simulink model "QuadcopterSimulationControl"  (R2016b)
settings: Solver=VariableStepAuto  StartTime=0.0  StopTime=100  RelTol=1e-3
values from neighbouring files (symbols this model uses):
  Ax = 0.1    [QuadcopterContants.m]
  Ay = 0.1    [QuadcopterContants.m]
  Az = 0.1    [QuadcopterContants.m]
  b = 1.144e-8    (= 1.144e-08)    [QuadcopterContants.m]
  d = 9.94e-10    [QuadcopterContants.m]
  g = 9.81    [QuadcopterContants.m]
  Ixx = 4.856e-3    (= 0.004856)    [QuadcopterContants.m]
  Iyy = 4.856e-3    (= 0.004856)    [QuadcopterContants.m]
  Izz = 8.801e-3    (= 0.008801)    [QuadcopterContants.m]
  Jr = 3.357e-5    (= 3.357e-05)    [QuadcopterContants.m]
  K_phi_D = 1    [QuadcopterContants.m]
  K_phi_I = 1    [QuadcopterContants.m]
  K_phi_p = 1    [QuadcopterContants.m]
  K_psi_D = 1    [QuadcopterContants.m]
  K_psi_I = 1    [QuadcopterContants.m]
  K_psi_p = 1    [QuadcopterContants.m]
  K_theta_D = 1    [QuadcopterContants.m]
  K_theta_I = 1    [QuadcopterContants.m]
  K_theta_p = 1    [QuadcopterContants.m]
  K_z_D = 1    [QuadcopterContants.m]
  K_z_I = 1    [QuadcopterContants.m]
  K_z_p = 1    [QuadcopterContants.m]
  l = 0.225    [QuadcopterContants.m]
  m = 0.468    [QuadcopterContants.m]
settings Model: Creator=alexzongo  LastModifiedBy=alexzongo

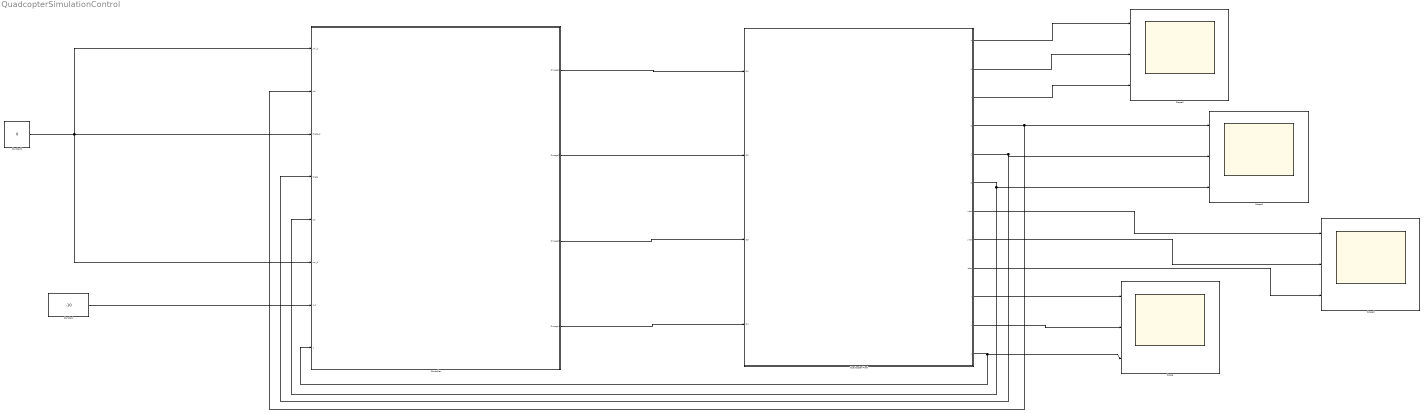
== system QuadcopterSimulationControl ==
  Constant : Constant  Value=-10
  Constant1 : Constant  Value=0
  Controller : Subsystem
  Quadcopter Plant : Subsystem
  Scope{,1..3} (4 alike) : Scope  NumInputPorts=3
  wires:
  Quadcopter Plant/4(𝜙) -> Scope1/1, Controller/2(phi)
  Quadcopter Plant/5("𝜃 ") -> Scope1/2, Controller/4(theta)
  Quadcopter Plant/6(𝜓) -> Scope1/3, Controller/5(psi)
  Quadcopter Plant/12(z) -> Scope/3, Controller/8(z)
  Controller/1(Omega1) -> Quadcopter Plant/1(Ω1)
  Controller/2(Omega2) -> Quadcopter Plant/2("Ω2 ")
  Controller/3(Omega3) -> Quadcopter Plant/3(Ω3)
  Controller/4(Omega4) -> Quadcopter Plant/4(Ω4)
  Constant1/1 -> Controller/6(psi_d), Controller/1(phi_d), Controller/3(theta_d)
  Constant/1 -> Controller/7(z_d)
  Quadcopter Plant/10(x) -> Scope/1
  Quadcopter Plant/11(y) -> Scope/2
  Quadcopter Plant/1(p) -> Scope2/1
  Quadcopter Plant/2(q) -> Scope2/2
  Quadcopter Plant/3(r) -> Scope2/3
  Quadcopter Plant/7(xdot) -> Scope3/1
  Quadcopter Plant/8(ydot) -> Scope3/2
  Quadcopter Plant/9(zdot) -> Scope3/3

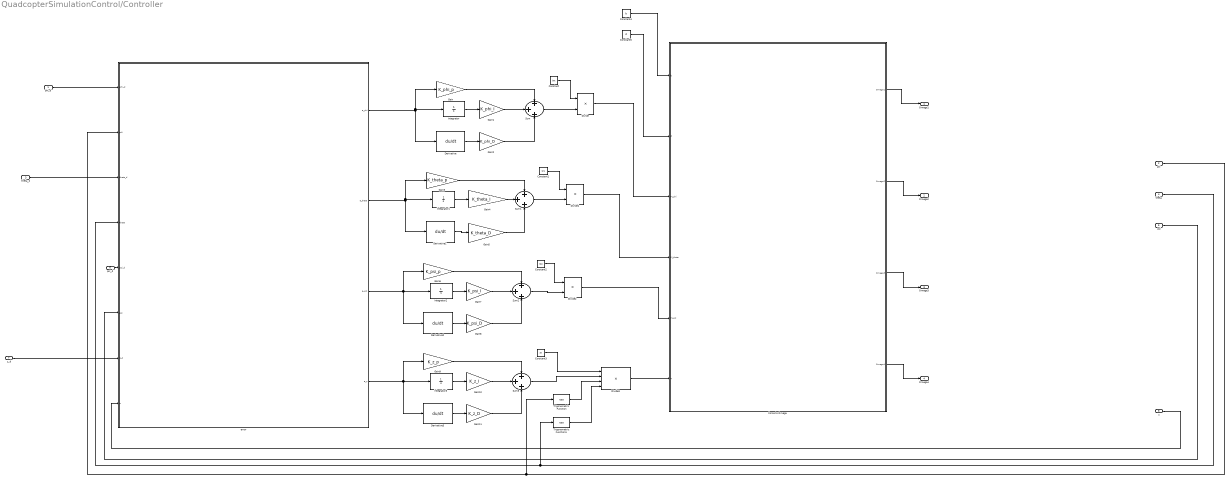
== system QuadcopterSimulationControl/Controller ==
  phi_d : Inport
  phi : Inport  Port=2
  theta_d : Inport  Port=3
  theta : Inport  Port=4
  psi : Inport  Port=5
  psi_d : Inport  Port=6
  z_d : Inport  Port=7
  z : Inport  Port=8
  Constant : Constant  Value=Ixx
  Constant1 : Constant  Value=Iyy
  Constant2 : Constant  Value=Izz
  Constant3 : Constant  Value=m
  Constant4 : Constant  Value=b
  Constant5 : Constant  Value=d
  Derivative{,1..3} (4 alike) : Derivative  CoefficientInTFapproximation=0
  Divide : Product  Inputs=**
  Divide1 : Product  Inputs=**
  Divide2 : Product  Inputs=**
  Divide3 : Product  Inputs=****
  Force to Omega : MATLAB Function  TreatAsAtomicUnit=on
  Gain : Gain  Gain=K_phi_p
  Gain1 : Gain  Gain=K_phi_I
  Gain10 : Gain  Gain=K_z_I
  Gain11 : Gain  Gain=K_z_D
  Gain2 : Gain  Gain=K_phi_D
  Gain3 : Gain  Gain=K_theta_p
  Gain4 : Gain  Gain=K_theta_I
  Gain5 : Gain  Gain=K_theta_D
  Gain6 : Gain  Gain=K_psi_p
  Gain7 : Gain  Gain=K_psi_I
  Gain8 : Gain  Gain=K_psi_D
  Gain9 : Gain  Gain=K_z_p
  Integrator{,1..3} (4 alike) : Integrator
  Sum{,1..3} (4 alike) : Sum  Inputs=+++
  Trigonometric Function : Trigonometry  Operator=cos
  Trigonometric Function1 : Trigonometry  Operator=cos
  error : MATLAB Function  TreatAsAtomicUnit=on
  Omega1 : Outport
  Omega2 : Outport  Port=2
  Omega3 : Outport  Port=3
  Omega4 : Outport  Port=4
  wires:
  Constant2/1 -> Divide2/1
  Divide2/1 -> Force to Omega/5(M_psi)
  Gain8/1 -> Sum2/3
  Constant3/1 -> Divide3/1
  Divide3/1 -> Force to Omega/6(T)
  Gain7/1 -> Sum2/2
  Sum2/1 -> Divide2/2
  Gain6/1 -> Sum2/1
  Derivative3/1 -> Gain11/1
  Gain10/1 -> Sum3/2
  Sum3/1 -> Divide3/2
  Gain11/1 -> Sum3/3
  Force to Omega/1(Omega1) -> Omega1/1
  Gain9/1 -> Sum3/1
  Force to Omega/4(Omega4) -> Omega4/1
  z_d/1 -> error/7(z_d)
  Derivative/1 -> Gain2/1
  Integrator/1 -> Gain1/1
  Divide/1 -> Force to Omega/3(M_phi)
  theta_d/1 -> error/3(theta_d)
  Gain1/1 -> Sum/2
  Gain/1 -> Sum/1
  error/1(e_phi) -> Derivative/1, Gain/1, Integrator/1
  phi/1 -> Trigonometric Function/1, error/2(phi)
  Trigonometric Function1/1 -> Divide3/4
  psi/1 -> error/6(psi)
  phi_d/1 -> error/1(phi_d)
  theta/1 -> Trigonometric Function1/1, error/4(theta)
  error/3(e_psi) -> Derivative2/1, Gain6/1, Integrator2/1
  Integrator2/1 -> Gain7/1
  Gain2/1 -> Sum/3
  error/2(e_theta) -> Derivative1/1, Gain3/1, Integrator1/1
  Divide1/1 -> Force to Omega/4(M_theta)
  error/4(e_z) -> Derivative3/1, Gain9/1, Integrator3/1
  Constant1/1 -> Divide1/1
  Integrator3/1 -> Gain10/1
  Gain5/1 -> Sum1/3
  Sum1/1 -> Divide1/2
  Derivative1/1 -> Gain5/1
  psi_d/1 -> error/5(psi_d)
  Force to Omega/3(Omega3) -> Omega3/1
  Force to Omega/2(Omega2) -> Omega2/1
  Gain3/1 -> Sum1/1
  Trigonometric Function/1 -> Divide3/3
  Gain4/1 -> Sum1/2
  Integrator1/1 -> Gain4/1
  Derivative2/1 -> Gain8/1
  Constant/1 -> Divide/1
  z/1 -> error/8(z)
  Sum/1 -> Divide/2
  Constant4/1 -> Force to Omega/1(b)
  Constant5/1 -> Force to Omega/2(d)

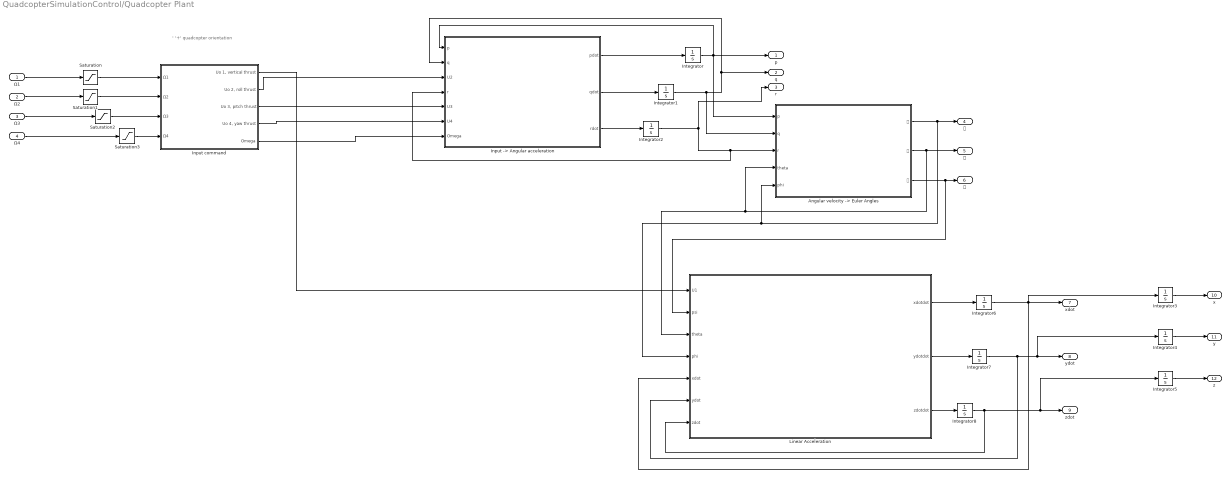
== system QuadcopterSimulationControl/Quadcopter Plant ==
  note: ' '+' quadcopter orientation
  Ω1 : Inport
  "Ω2 " : Inport  Port=2
  Ω3 : Inport  Port=3
  Ω4 : Inport  Port=4
  "Angular velocity -> Euler Angles" : Subsystem
  "Input -> Angular acceleration" : Subsystem
  "Input command " : Subsystem
  Integrator{,1..2,6..8} (6 alike) : Integrator
  Integrator3 : Integrator  LimitOutput=on
  Integrator4 : Integrator  LimitOutput=on
  Integrator5 : Integrator  LimitOutput=on  UpperSaturationLimit=0
  Linear Acceleration : Subsystem
  Saturation{,1..3} (4 alike) : Saturate  UpperLimit=inf  LowerLimit=0
  p : Outport
  q : Outport  Port=2
  r : Outport  Port=3
  𝜙 : Outport  Port=4
  "𝜃 " : Outport  Port=5
  𝜓 : Outport  Port=6
  xdot : Outport  Port=7
  ydot : Outport  Port=8
  zdot : Outport  Port=9
  x : Outport  Port=10
  y : Outport  Port=11
  z : Outport  Port=12
  wires:
  Ω1/1 -> Saturation/1
  "Ω2 "/1 -> Saturation1/1
  Ω3/1 -> Saturation2/1
  Ω4/1 -> Saturation3/1
  "Input command "/1("Uo 1, vertical thrust") -> Linear Acceleration/1(U1)
  Integrator/1 -> "Angular velocity -> Euler Angles"/1(p), "Input -> Angular acceleration"/1(p), p/1
  Integrator1/1 -> q/1, "Input -> Angular acceleration"/2(q), "Angular velocity -> Euler Angles"/2(q)
  Integrator2/1 -> r/1, "Input -> Angular acceleration"/4(r), "Angular velocity -> Euler Angles"/3(r)
  Integrator8/1 -> Integrator5/1, zdot/1, Linear Acceleration/7(zdot)
  Integrator7/1 -> Linear Acceleration/6(ydot), Integrator4/1, ydot/1
  Integrator6/1 -> Integrator3/1, Linear Acceleration/5(xdot), xdot/1
  "Input command "/2("Uo 2, roll thrust") -> "Input -> Angular acceleration"/3(U2)
  "Input command "/3("Uo 3, pitch thrust") -> "Input -> Angular acceleration"/5(U3)
  "Input command "/5(Omega) -> "Input -> Angular acceleration"/7(Omega)
  "Input -> Angular acceleration"/1(pdot) -> Integrator/1
  "Input -> Angular acceleration"/2(qdot) -> Integrator1/1
  "Input -> Angular acceleration"/3(rdot) -> Integrator2/1
  "Angular velocity -> Euler Angles"/3(𝜓) -> Linear Acceleration/2(psi), 𝜓/1
  "Angular velocity -> Euler Angles"/1(𝜙) -> Linear Acceleration/4(phi), "Angular velocity -> Euler Angles"/5(phi), 𝜙/1
  "Angular velocity -> Euler Angles"/2(𝜃) -> Linear Acceleration/3(theta), "Angular velocity -> Euler Angles"/4(theta), "𝜃 "/1
  Linear Acceleration/1(xdotdot) -> Integrator6/1
  Linear Acceleration/2(ydotdot) -> Integrator7/1
  Linear Acceleration/3(zdotdot) -> Integrator8/1
  Integrator3/1 -> x/1
  Integrator4/1 -> y/1
  Integrator5/1 -> z/1
  Saturation/1 -> "Input command "/1(Ω1)
  Saturation1/1 -> "Input command "/2("Ω2 ")
  Saturation2/1 -> "Input command "/3(Ω3)
  Saturation3/1 -> "Input command "/4(Ω4)
  "Input command "/4("Uo 4, yaw thrust") -> "Input -> Angular acceleration"/6(U4)

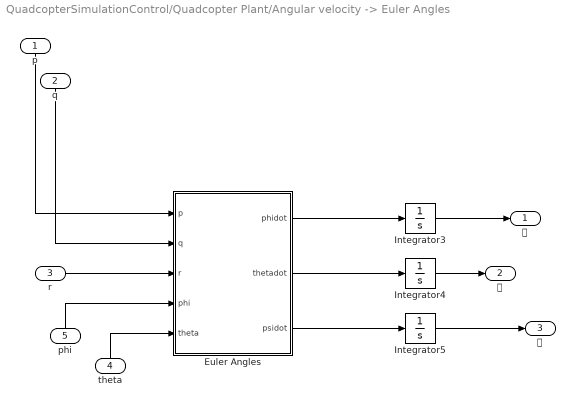
== system QuadcopterSimulationControl/Quadcopter Plant/Angular velocity -> Euler Angles ==
  p : Inport
  q : Inport  Port=2
  r : Inport  Port=3
  theta : Inport  Port=4
  phi : Inport  Port=5
  Euler Angles : MATLAB Function  TreatAsAtomicUnit=on
  Integrator3 : Integrator  WrapState=on
  Integrator4 : Integrator  WrapState=on
  Integrator5 : Integrator  WrapState=on
  𝜙 : Outport
  𝜃 : Outport  Port=2
  𝜓 : Outport  Port=3
  wires:
  theta/1 -> Euler Angles/5(theta)
  p/1 -> Euler Angles/1(p)
  phi/1 -> Euler Angles/4(phi)
  q/1 -> Euler Angles/2(q)
  r/1 -> Euler Angles/3(r)
  Euler Angles/3(psidot) -> Integrator5/1
  Integrator3/1 -> 𝜙/1
  Euler Angles/2(thetadot) -> Integrator4/1
  Integrator5/1 -> 𝜓/1
  Euler Angles/1(phidot) -> Integrator3/1
  Integrator4/1 -> 𝜃/1

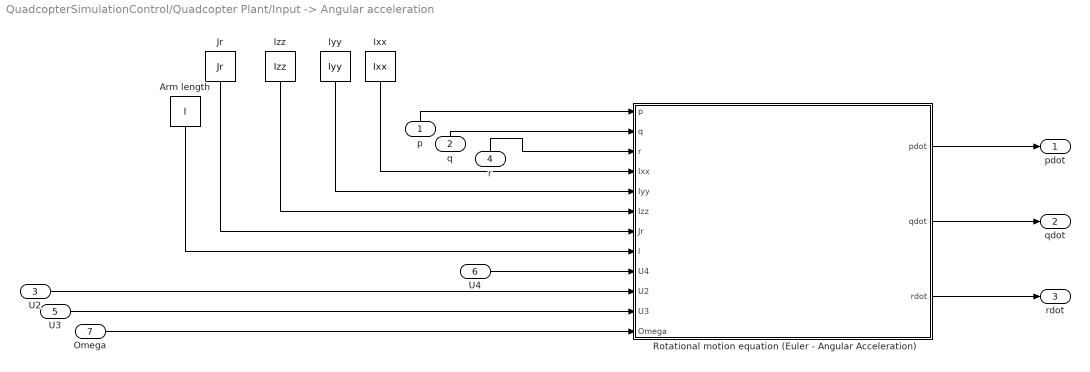
== system QuadcopterSimulationControl/Quadcopter Plant/Input -> Angular acceleration ==
  p : Inport
  q : Inport  Port=2
  U2 : Inport  Port=3
  r : Inport  Port=4
  U3 : Inport  Port=5
  U4 : Inport  Port=6
  Omega : Inport  Port=7
  "Arm length " : Constant  Value=l
  Ixx : Constant  Value=Ixx
  Iyy : Constant  Value=Iyy
  Izz : Constant  Value=Izz
  Jr : Constant  Value=Jr
  Rotational motion equation (Euler - Angular Acceleration) : MATLAB Function  TreatAsAtomicUnit=on
  pdot : Outport
  qdot : Outport  Port=2
  rdot : Outport  Port=3
  wires:
  U4/1 -> Rotational motion equation (Euler - Angular Acceleration)/9(U4)
  p/1 -> Rotational motion equation (Euler - Angular Acceleration)/1(p)
  q/1 -> Rotational motion equation (Euler - Angular Acceleration)/2(q)
  r/1 -> Rotational motion equation (Euler - Angular Acceleration)/3(r)
  Ixx/1 -> Rotational motion equation (Euler - Angular Acceleration)/4(Ixx)
  Izz/1 -> Rotational motion equation (Euler - Angular Acceleration)/6(Izz)
  Iyy/1 -> Rotational motion equation (Euler - Angular Acceleration)/5(Iyy)
  Jr/1 -> Rotational motion equation (Euler - Angular Acceleration)/7(Jr)
  "Arm length "/1 -> Rotational motion equation (Euler - Angular Acceleration)/8(l)
  Omega/1 -> Rotational motion equation (Euler - Angular Acceleration)/12(Omega)
  U3/1 -> Rotational motion equation (Euler - Angular Acceleration)/11(U3)
  U2/1 -> Rotational motion equation (Euler - Angular Acceleration)/10(U2)
  Rotational motion equation (Euler - Angular Acceleration)/1(pdot) -> pdot/1
  Rotational motion equation (Euler - Angular Acceleration)/2(qdot) -> qdot/1
  Rotational motion equation (Euler - Angular Acceleration)/3(rdot) -> rdot/1

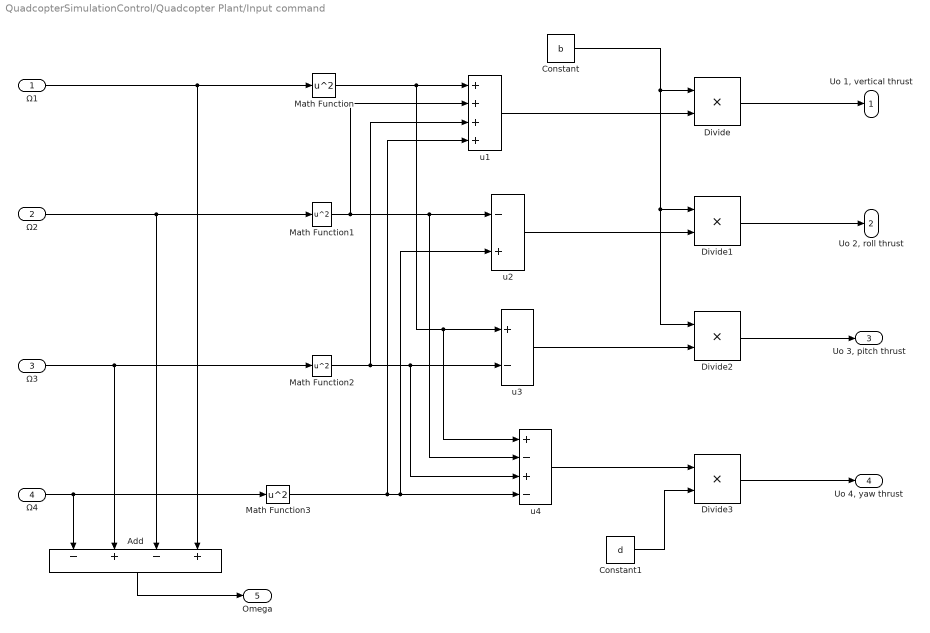
== system QuadcopterSimulationControl/Quadcopter Plant/Input command  ==
  Ω1 : Inport
  "Ω2 " : Inport  Port=2
  Ω3 : Inport  Port=3
  Ω4 : Inport  Port=4
  Add : Sum  Inputs=-+-+
  Constant : Constant  Value=b
  Constant1 : Constant  Value=d
  Divide{,1..3} (4 alike) : Product
  Math Function{,1..3} (4 alike) : Math  Operator=square  SaturateOnIntegerOverflow=on
  u1 : Sum  Inputs=4
  u2 : Sum  Inputs=-+
  u3 : Sum  Inputs=+-
  u4 : Sum  Inputs=+-+-
  "Uo 1, vertical thrust" : Outport
  "Uo 2, roll thrust" : Outport  Port=2
  "Uo 3, pitch thrust" : Outport  Port=3
  "Uo 4, yaw thrust" : Outport  Port=4
  Omega : Outport  Port=5
  wires:
  Ω4/1 -> Add/1, Math Function3/1
  Ω3/1 -> Add/2, Math Function2/1
  "Ω2 "/1 -> Add/3, Math Function1/1
  Ω1/1 -> Add/4, Math Function/1
  Add/1 -> Omega/1
  Math Function/1 -> u4/1, u3/1, u1/1
  Math Function1/1 -> u4/2, u2/1, u1/2
  Math Function2/1 -> u4/3, u3/2, u1/3
  Math Function3/1 -> u4/4, u2/2, u1/4
  Constant/1 -> Divide/1, Divide2/1, Divide1/1
  u1/1 -> Divide/2
  Constant1/1 -> Divide3/2
  u4/1 -> Divide3/1
  u3/1 -> Divide2/2
  u2/1 -> Divide1/2
  Divide/1 -> "Uo 1, vertical thrust"/1
  Divide1/1 -> "Uo 2, roll thrust"/1
  Divide2/1 -> "Uo 3, pitch thrust"/1
  Divide3/1 -> "Uo 4, yaw thrust"/1

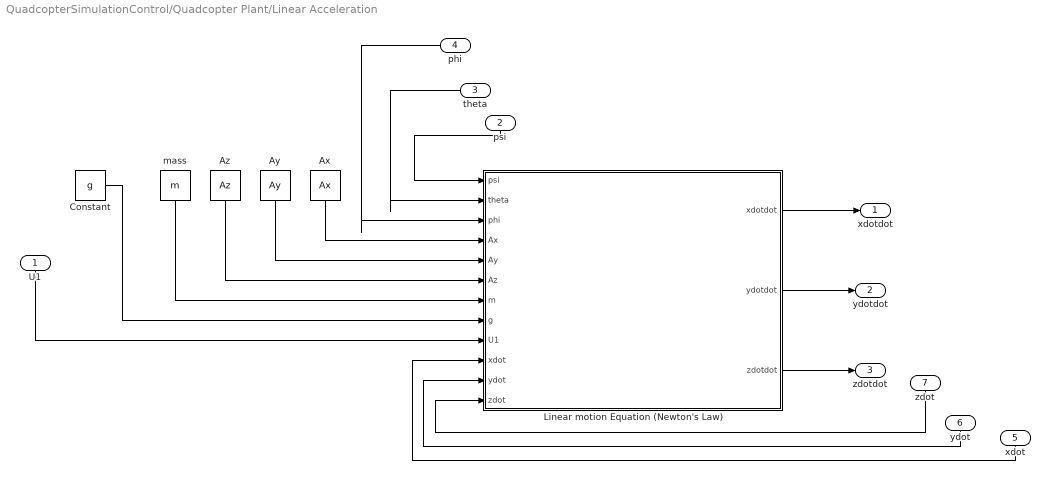
== system QuadcopterSimulationControl/Quadcopter Plant/Linear Acceleration ==
  U1 : Inport
  psi : Inport  Port=2
  theta : Inport  Port=3
  phi : Inport  Port=4
  xdot : Inport  Port=5
  ydot : Inport  Port=6
  zdot : Inport  Port=7
  Ax : Constant  Value=Ax
  Ay : Constant  Value=Ay
  Az : Constant  Value=Az
  Constant : Constant  Value=g
  Linear motion Equation (Newton's Law) : MATLAB Function  TreatAsAtomicUnit=on
  mass : Constant  Value=m
  xdotdot : Outport
  ydotdot : Outport  Port=2
  zdotdot : Outport  Port=3
  wires:
  zdot/1 -> Linear motion Equation (Newton's Law)/12(zdot)
  theta/1 -> Linear motion Equation (Newton's Law)/2(theta)
  psi/1 -> Linear motion Equation (Newton's Law)/1(psi)
  U1/1 -> Linear motion Equation (Newton's Law)/9(U1)
  xdot/1 -> Linear motion Equation (Newton's Law)/10(xdot)
  phi/1 -> Linear motion Equation (Newton's Law)/3(phi)
  ydot/1 -> Linear motion Equation (Newton's Law)/11(ydot)
  Linear motion Equation (Newton's Law)/3(zdotdot) -> zdotdot/1
  Ax/1 -> Linear motion Equation (Newton's Law)/4(Ax)
  Az/1 -> Linear motion Equation (Newton's Law)/6(Az)
  mass/1 -> Linear motion Equation (Newton's Law)/7(m)
  Ay/1 -> Linear motion Equation (Newton's Law)/5(Ay)
  Linear motion Equation (Newton's Law)/1(xdotdot) -> xdotdot/1
  Linear motion Equation (Newton's Law)/2(ydotdot) -> ydotdot/1
  Constant/1 -> Linear motion Equation (Newton's Law)/8(g)

== matlab function QuadcopterSimulationControl/Quadcopter Plant/Angular velocity -> Euler Angles/Euler Angles ==
  data: p input; phidot output; q input; r input; phi input; theta input; thetadot output; psidot output
function [phidot, thetadot, psidot] = fcn(p, q, r, phi, theta)

R = [1 sin(phi)*tan(theta) cos(phi)*tan(theta);
     0 cos(phi) -sin(phi);
     0 sin(phi)/cos(theta) cos(phi)/cos(theta)];
Phi = R*[p;q;r];
phidot = Phi(1);
thetadot = Phi(2);
psidot = Phi(3);

== matlab function QuadcopterSimulationControl/Quadcopter Plant/Input -> Angular acceleration/Rotational motion equation (Euler - Angular Acceleration) ==
  data: p input; q input; r input; Ixx input; pdot output; Iyy input; Izz input; Jr input; l input; U4 input; U2 input; U3 input; Omega input; qdot output; rdot output
function [pdot, qdot, rdot] = fcn(p, q, r, Ixx, Iyy, Izz, Jr, l, U4, U2,U3, Omega)
    
pdot = (Iyy-Izz)*q*r/Ixx - Jr*q*Omega/Ixx + l*U2/Ixx;
qdot = (Izz-Ixx)*p*r/Iyy - Jr*p*Omega/Iyy + l*U3/Iyy;
rdot = (Ixx-Iyy)*q*p/Izz + U4/Izz;

== matlab function QuadcopterSimulationControl/Quadcopter Plant/Linear Acceleration/Linear motion Equation (Newton's Law) ==
  data: psi input; theta input; phi input; Ax input; Ay input; Az input; m input; g input; U1 input; xdotdot output; xdot input; ydot input; zdot input; ydotdot output; zdotdot output
function [xdotdot, ydotdot, zdotdot] = fcn(psi, theta, phi, Ax, Ay, Az, m, g, U1, xdot, ydot, zdot)

xdotdot = ((sin(phi)*sin(psi) - cos(psi)*sin(theta)*cos(phi))*U1 - Ax*xdot)/m;
ydotdot = ((sin(phi)*cos(psi) + sin(psi)*sin(theta)*cos(phi))*U1 - Ay*ydot)/m;
zdotdot = (m*g - (cos(theta)*cos(phi))*U1 - Az*zdot)/m;

== matlab function QuadcopterSimulationControl/Controller/error ==
  data: phi_d input; e_phi output; phi input; theta_d input; theta input; psi_d input; psi input; z_d input; z input; e_theta output; e_psi output; e_z output
function [e_phi, e_theta, e_psi, e_z] = fcn(phi_d, phi, theta_d, theta, psi_d, psi, z_d, z)

 e_phi = phi_d-phi;
 e_theta = theta_d-theta;
 e_psi = psi_d-psi;
 e_z = z_d - z;

== matlab function QuadcopterSimulationControl/Controller/Force to Omega ==
  data: b input; d input; M_phi input; Omega1 output; M_theta input; M_psi input; T input; Omega2 output; Omega3 output; Omega4 output
function [Omega1, Omega2, Omega3, Omega4] = fcn(b, d, M_phi, M_theta, M_psi, T)

F = [T M_phi M_theta M_psi]';
M = [1/(4*b) 0 1/(2*b) 1/(4*d);
     1/(4*b) -1/(2*b) 0 -1/(4*d);
     1/(4*b) 0 -1/(2*b) -1/(4*d);
     1/(4*b) 1/(2*b) 0 -1/(4*d)];

Omega_square = M*F;

Omega1 = sqrt(abs(Omega_square(1)));
Omega2 = sqrt(abs(Omega_square(2)));
Omega3 = sqrt(abs(Omega_square(3)));
Omega4 = sqrt(abs(Omega_square(4)));
